simulink model "halfcar_seat"  (R2024a)
settings: Solver=FixedStepAuto  StartTime=0.0  StopTime=15  FixedStep=0.001  RelTol=1e-3
values from neighbouring files (symbols this model uses):
  A = [0            0           0                     0                           0           1           0                     0                                  0                                  0 ... (first row only)    [half_suspension_final.m]
  B = [0      0 ... (first row only)    [half_suspension_final.m]
  C = [0 0 1 0 0 0 0 0 0 0 ... (first row only)    [half_suspension_final.m]
  D = [0 0 ... (first row only)    [half_suspension_final.m]
libraries: simulink_extras x1
settings Model: Creator=cop23agk  LastModifiedBy=cop23agk

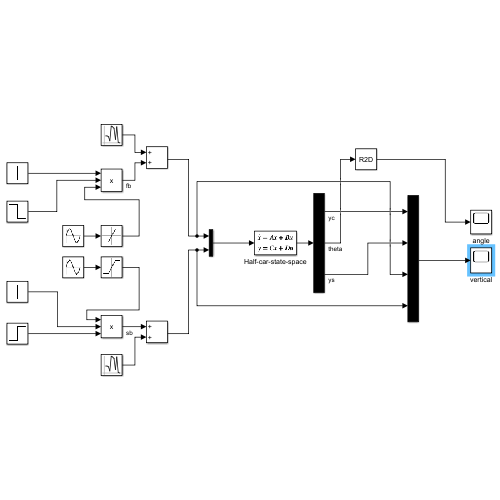
[thumbnail: Simulink's stored preview of the top-level diagram]
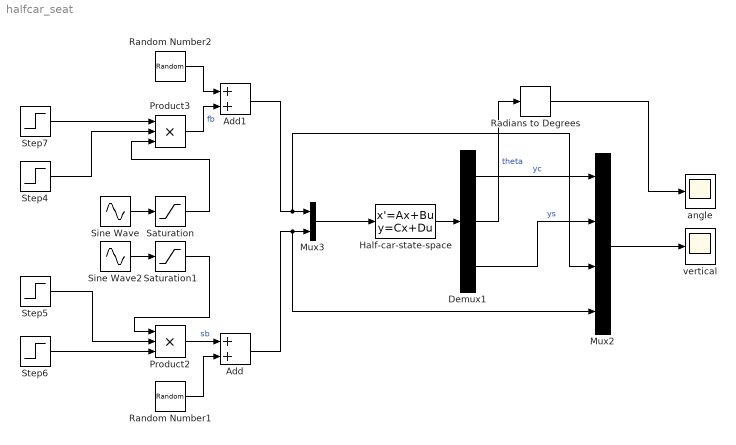
== system halfcar_seat ==
  Add : Sum
  Add1 : Sum
  Demux1 : Demux  Outputs=3
  Half-car-state-space : StateSpace  A=A  B=B  C=C  D=D  InitialCondition=0
  Mux2 : Mux
  Mux3 : Mux  Inputs=2
  Product2 : Product  Inputs=3
  Product3 : Product  Inputs=3
  Radians to Degrees : simulink_extras/Transformations/Radians to Degrees
  Random Number1 : RandomNumber  Variance=0.000001  SampleTime=0
  Random Number2 : RandomNumber  Variance=0.000001  SampleTime=0
  Saturation : Saturate  LowerLimit=0
  Saturation1 : Saturate  LowerLimit=0
  Sine Wave : Sin  Amplitude=0.1  Frequency=3.14159265  SampleTime=0
  Sine Wave2 : Sin  Amplitude=0.1  Frequency=3.14159265  Phase=2*pi  SampleTime=0
  Step4 : Step  Time=3.5  Before=1  After=0  SampleTime=0
  Step5 : Step  Time=5.5  Before=1  After=0  SampleTime=0
  Step6 : Step  Time=3.5  SampleTime=0
  Step7 : Step  Time=1.5  SampleTime=0
  angle : Scope
  vertical : Scope
  wires:
  Demux1/1 -> Mux2/1  "yc"
  Mux2/1 -> vertical/1
  Mux3/1 -> Half-car-state-space/1
  Demux1/3 -> Mux2/2  "ys"
  Demux1/2 -> Radians to Degrees/1  "theta"
  Sine Wave/1 -> Saturation/1
  Sine Wave2/1 -> Saturation1/1
  Radians to Degrees/1 -> angle/1
  Step7/1 -> Product3/1
  Step4/1 -> Product3/2
  Saturation1/1 -> Product2/1
  Step6/1 -> Product2/3
  Random Number1/1 -> Add/2
  Product2/1 -> Add/1  "sb"
  Product3/1 -> Add1/2  "fb"
  Saturation/1 -> Product3/3
  Random Number2/1 -> Add1/1
  Step5/1 -> Product2/2
  Half-car-state-space/1 -> Demux1/1
  Add1/1 -> Mux2/3, Mux3/1
  Add/1 -> Mux2/4, Mux3/2
